simulink model "rlWalkingspotmini_ly"  (R2019a)
settings: Solver=ode113  StartTime=0.0  StopTime=Tf  FixedStep=0.025  RelTol=1e-1  EnableMultiTasking=on
values from neighbouring files (symbols this model uses):
  Tf = 10    [initializeRobotParameters.m]
  Ts = 0.025    [initializeRobotParameters.m]
undefined symbols (not defined in the file or in its folder): height_plane, init_angs_R, init_height, joint_stiffness, plane_x, plane_y, wx0, wy0, X, Y, Z
libraries: sm_lib x66, rlWalkingRobotUtils x20, nesl_utility x14, simulink x5, rllib x1, robotcorelib x1
(part 3 of 3)

== system rlWalkingspotmini_ly/Walking Robot/Sensors/Calculate Actuator Power3 ==
  meas : Inport
  Add : Sum  Inputs=3
  Bus Selector : BusSelector  OutputSignals=ankle_speed,ankle_torque,knee_speed,knee_torque,hip_speed,hip_torque
  Product : Product
  Product1 : Product
  Product2 : Product
  P : Outport
  wires:
  meas/1 -> Bus Selector/1
  Product2/1 -> Add/3
  Product1/1 -> Add/2
  Product/1 -> Add/1
  Add/1 -> P/1
  Bus Selector/1 -> Product/1  "<ankle_speed>"
  Bus Selector/2 -> Product/2  "<ankle_torque>"
  Bus Selector/3 -> Product1/1  "<knee_speed>"
  Bus Selector/4 -> Product1/2  "<knee_torque>"
  Bus Selector/5 -> Product2/1  "<hip_speed>"
  Bus Selector/6 -> Product2/2  "<hip_torque>"
